simulink model "simulation_model"  (R2022a)
settings: Solver=VariableStepAuto  StartTime=0.0  StopTime=inf  FixedStep=0.02  MaxStep=0.1  RelTol=1e-3
values from neighbouring files (symbols this model uses):
  psi0 = atan(yc/xc)    [close_example.m]    (also in example_m.m)
  xc = coordinate(1)    [close_example.m]    (also in example_m.m)
  yc = coordinate(2)    [close_example.m]    (also in example_m.m)
undefined symbols (not defined in the file or in its folder): fuel_rate, gamma_pb, Pose, sigbuilder_block
libraries: simulink_extras x4, robotlib x3, simulink x1
(part 1 of 3)
settings Model: Creator=Rafal  LastModifiedBy=offroad
settings OptimizationCC: DefaultParameterBehavior=Inlined  EnhancedBackFolding=on  PassReuseOutputArgsAs=Individual arguments  ZeroExternalMemoryAtStartup=off  ZeroInternalMemoryAtStartup=off  MaxStackSize=64  OptimizeBlockOrder=speed  DifferentSizesBufferReuse=on  OptimizationCustomize=off  EfficientTunableParamExpr=on
settings DebuggingCC: ParameterTunabilityLossMsg=error
settings HardwareCC: ProdBitPerPointer=32  ProdBitPerSizeT=32  ProdBitPerPtrDiffT=32  ProdLargestAtomicFloat=None  ProdIntDivRoundTo=Undefined  ProdEndianess=Unspecified  ProdWordSize=32  ProdHWDeviceType=Generic->Unspecified (assume 32-bit Generic)  UseEmbeddedCoderFeatures=off
settings SFSimCC: MATLABDynamicMemAlloc=off
settings RTWCC: SystemTargetFile=ert.tlc  TemplateMakefile=ert_default_tmf  Toolchain=Catkin
settings CodeAppCC: ForceParamTrailComments=on  IgnoreCustomStorageClasses=off  OperatorAnnotations=on  SimulinkDataObjDesc=on  SFDataObjDesc=on  InsertBlockDesc=on
settings ERTTargetCC: SupportNonInlinedSFcns=on  ERTCustomFileTemplate=example_file_process.tlc

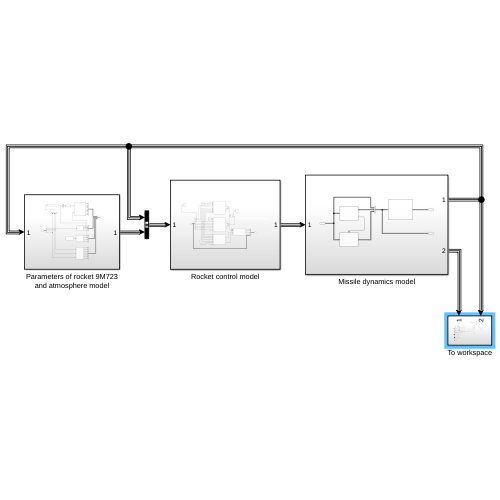
[thumbnail: Simulink's stored preview of the top-level diagram]
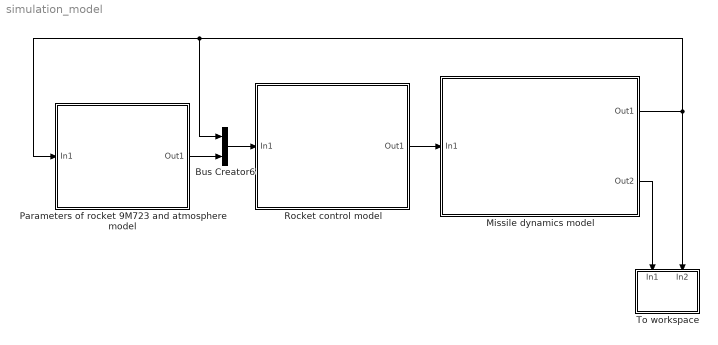
== system simulation_model ==
  Bus Creator6 : BusCreator  Inputs=2
  Missile dynamics model : Subsystem
  Parameters of rocket 9M723 and atmosphere model : Subsystem
  Rocket control model : Subsystem
  To workspace : Subsystem
  wires:
  Bus Creator6/1 -> Rocket control model/1(In1)
  Parameters of rocket 9M723 and atmosphere model/1(Out1) -> Bus Creator6/2
  Missile dynamics model/1(Out1) -> To workspace/2(In2), Parameters of rocket 9M723 and atmosphere model/1(In1), Bus Creator6/1
  Missile dynamics model/2(Out2) -> To workspace/1(In1)
  Rocket control model/1(Out1) -> Missile dynamics model/1(In1)

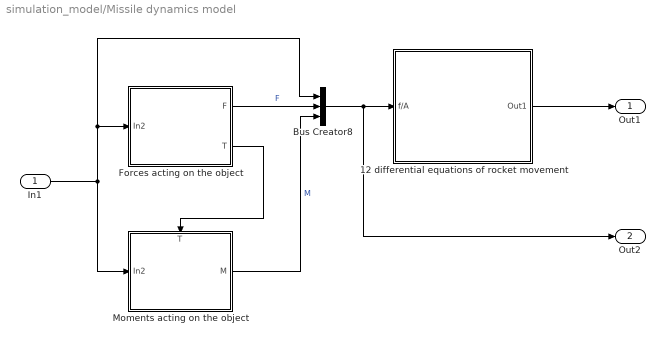
== system simulation_model/Missile dynamics model ==
  In1 : Inport
  "12 differential equations of rocket movement " : Subsystem
  Bus Creator8 : BusCreator  Inputs=3
  "Forces acting on the object " : Subsystem
  Moments acting on the object : Subsystem
      settings: PortSchema="{\"entries\":[{\"content\":{\"sides\":[{\"content\":{\"connectorIds\":[\"In1\"]},\"type\":\"ConnectorPlacement.EquallySpacedRectSide\",\"uuid\":\"23a5d515-3fe3-43ba-a5a2-a9cfb4131548\"},{\"content\":{\"connectorIds\":[\"Out1\"],\"side\":\"RIGHT\"},\"type\":\"ConnectorPlacement.EquallySpacedRectSide\",\"uuid\":\"38b37899-0e98-470d-b21c-2ca9e40fcf87\"},{\"content\":{\"connectorIds\":[\"In2\"],\"side\":\"TOP\"},\"type\":\"ConnectorPlacement.EquallySpacedRectSide\",\"uuid\":\"7a45db12-7300-424e-9c7b-41707e33aad7\"}]},\"type\":\"ConnectorPlacement.EquallySpacedConnector\",\"uuid\":\"8f829a99-de5c-4ee4-a55c-0d0490bb16ea\"}],\"packageUris\":[\"http://schema.mathworks.com/mf0/Connector/R2020b\"],\"version\":\"1.0\"}"
  Out1 : Outport
  Out2 : Outport  Port=2
  wires:
  In1/1 -> Bus Creator8/1, "Forces acting on the object "/1(In2), Moments acting on the object/1(In2)
  Bus Creator8/1 -> Out2/1, "12 differential equations of rocket movement "/1(f/A)
  Moments acting on the object/1(M) -> Bus Creator8/3  "M"
  "Forces acting on the object "/2(T) -> Moments acting on the object/2(T)
  "Forces acting on the object "/1(F) -> Bus Creator8/2  "F"
  "12 differential equations of rocket movement "/1(Out1) -> Out1/1

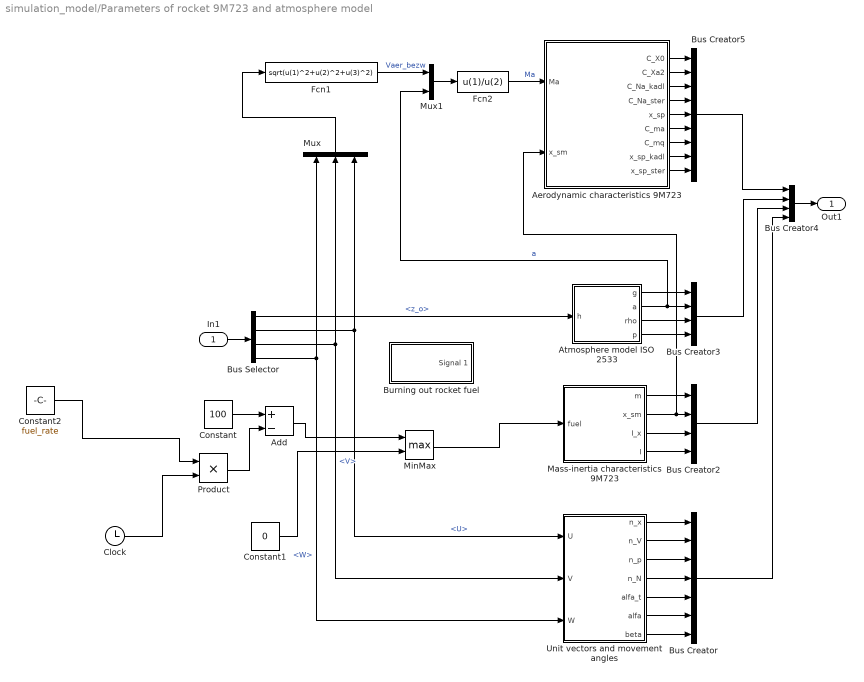
== system simulation_model/Parameters of rocket 9M723 and atmosphere model ==
  In1 : Inport
  Add : Sum  Inputs=+-
  Aerodynamic characteristics 9M723 : MATLAB Function  TreatAsAtomicUnit=on
  Atmosphere model ISO 2533 : MATLAB Function  TreatAsAtomicUnit=on
  Burning out rocket fuel : Subsystem  Tag=STV Subsys  LoadFcn=sigbuilder_block('load');  StartFcn=sigbuilder_block('start');  StopFcn=sigbuilder_block('stop');  ClipboardFcn=sigbuilder_block('clipboard');  mask(Sigbuilder block){tuvar=[0:10]}
      mask help: Simulink:masks:SigbuilderBlock_MD
      mask init:
      | if ~strcmp(get_param(bdroot(gcbh),'SimulationStatus'),'stopped') tuvar = sigbuilder_block('maskInit'); end
      settings: CopyFcn=sigbuilder_block('copy');  DeleteFcn=sigbuilder_block('delete');  ModelCloseFcn=sigbuilder_block('modelClose');  PreSaveFcn=sigbuilder_block('preSave');  PauseFcn=sigbuilder_block('pause');  ContinueFcn=sigbuilder_block('continue');  NameChangeFcn=sigbuilder_block('namechange');  OpenFcn=sigbuilder_block('open',[525 156.75 603 363.75 ]);  CloseFcn=sigbuilder_block('close');
      mask Display: plot(0, 0, 100, 100,[2, 2, 32, 32, 2], [68, 8, 8, 68, 68],[32, 2], [38, 38], [32, 19, 2],[53, 60, 44], [32, 17, 17, 2],[16, 16, 31, 31]);txt = getActiveGroup(gcbh);text(2, 100, txt,'verticalAlignment', 'top');
  Bus Creator : BusCreator  Inputs=7
  Bus Creator2 : BusCreator  Inputs=4
  Bus Creator3 : BusCreator  Inputs=4
  Bus Creator4 : BusCreator  Inputs=4
  Bus Creator5 : BusCreator  Inputs=9
  Bus Selector : BusSelector  OutputSignals=z_o,U,V,W
  Clock : Clock
  Constant : Constant  Value=100
  Constant1 : Constant  Value=0
  Constant2 : Constant  Value=fuel_rate
  Fcn1 : Fcn  Expr=sqrt(u(1)^2+u(2)^2+u(3)^2)
  Fcn2 : Fcn  Expr=u(1)/u(2)
  Mass-inertia characteristics 9M723 : MATLAB Function  TreatAsAtomicUnit=on
  MinMax : MinMax  Function=max  Inputs=2
  Mux : Mux  Inputs=3
  Mux1 : Mux  Inputs=2
  Product : Product
  Unit vectors and movement angles : MATLAB Function  TreatAsAtomicUnit=on
  Out1 : Outport
  wires:
  Aerodynamic characteristics 9M723/2(C_Xa2) -> Bus Creator5/2
  Aerodynamic characteristics 9M723/1(C_X0) -> Bus Creator5/1
  Bus Creator3/1 -> Bus Creator4/2
  Atmosphere model ISO 2533/2(a) -> Mux1/2, Bus Creator3/2  "a"
  Aerodynamic characteristics 9M723/5(x_sp) -> Bus Creator5/5
  Aerodynamic characteristics 9M723/4(C_Na_ster) -> Bus Creator5/4
  Aerodynamic characteristics 9M723/9(x_sp_ster) -> Bus Creator5/9
  Aerodynamic characteristics 9M723/8(x_sp_kadl) -> Bus Creator5/8
  Mass-inertia characteristics 9M723/3(I_x) -> Bus Creator2/3
  Bus Creator5/1 -> Bus Creator4/1
  Unit vectors and movement angles/4(n_N) -> Bus Creator/4
  Mux/1 -> Fcn1/1
  Aerodynamic characteristics 9M723/3(C_Na_kadl) -> Bus Creator5/3
  Mass-inertia characteristics 9M723/4(I) -> Bus Creator2/4
  Bus Creator/1 -> Bus Creator4/4
  Bus Selector/1 -> Atmosphere model ISO 2533/1(h)  "<z_o>"
  Bus Creator4/1 -> Out1/1
  Fcn1/1 -> Mux1/1  "Vaer_bezw"
  Unit vectors and movement angles/7(beta) -> Bus Creator/7
  Bus Selector/4 -> Mux/1, Unit vectors and movement angles/3(W)  "<W>"
  Atmosphere model ISO 2533/1(g) -> Bus Creator3/1
  Bus Selector/3 -> Mux/2, Unit vectors and movement angles/2(V)  "<V>"
  Unit vectors and movement angles/6(alfa) -> Bus Creator/6
  Unit vectors and movement angles/3(n_p) -> Bus Creator/3
  Unit vectors and movement angles/2(n_V) -> Bus Creator/2
  Unit vectors and movement angles/1(n_x) -> Bus Creator/1
  Unit vectors and movement angles/5(alfa_t) -> Bus Creator/5
  Bus Creator2/1 -> Bus Creator4/3
  Bus Selector/2 -> Unit vectors and movement angles/1(U), Mux/3  "<U>"
  Fcn2/1 -> Aerodynamic characteristics 9M723/1(Ma)  "Ma"
  Mass-inertia characteristics 9M723/1(m) -> Bus Creator2/1
  Mass-inertia characteristics 9M723/2(x_sm) -> Aerodynamic characteristics 9M723/2(x_sm), Bus Creator2/2
  Aerodynamic characteristics 9M723/6(C_ma) -> Bus Creator5/6
  Aerodynamic characteristics 9M723/7(C_mq) -> Bus Creator5/7
  Atmosphere model ISO 2533/4(p) -> Bus Creator3/4
  Mux1/1 -> Fcn2/1
  Atmosphere model ISO 2533/3(rho) -> Bus Creator3/3
  In1/1 -> Bus Selector/1
  Clock/1 -> Product/2
  Constant/1 -> Add/1
  Product/1 -> Add/2
  Add/1 -> MinMax/1
  Constant1/1 -> MinMax/2
  MinMax/1 -> Mass-inertia characteristics 9M723/1(fuel)
  Constant2/1 -> Product/1

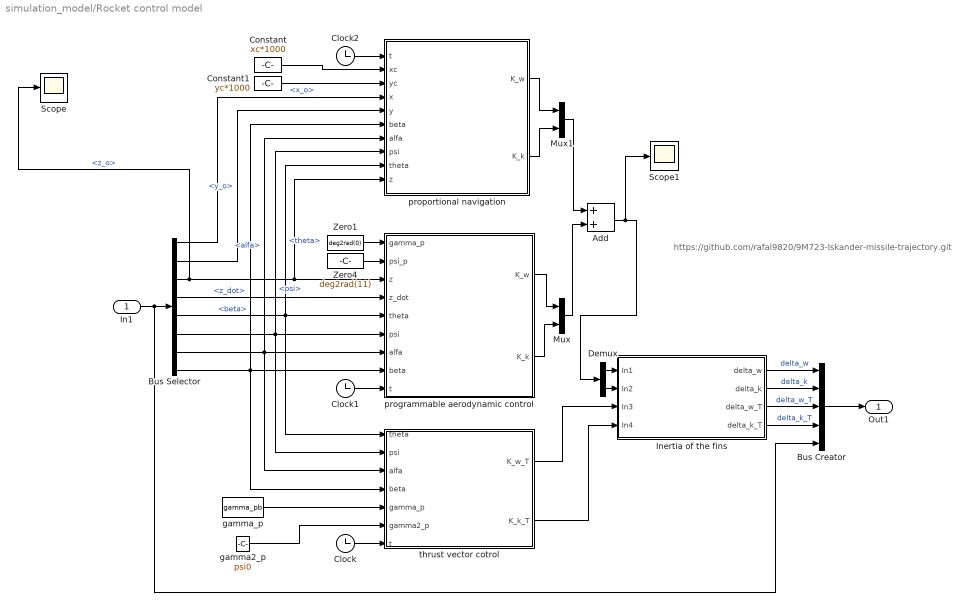
== system simulation_model/Rocket control model ==
  note: https://github.com/rafal9820/9M723-Iskander-missile-trajectory.git
  In1 : Inport
  Add : Sum
  Bus Creator : BusCreator  Inputs=5
  Bus Selector : BusSelector  OutputSignals=signal1.x_o,signal1.y_o,signal1.z_o,signal1.z_dot,signal1.theta,signal1.psi,signal2.signal4.alfa,signal2.signal4.beta
  Clock : Clock
  Clock1 : Clock
  Clock2 : Clock
  Constant : Constant  Value=xc*1000
  Constant1 : Constant  Value=yc*1000
  Demux : Demux  Outputs=2
  "Inertia of the fins " : Subsystem
  Mux : Mux  Inputs=2
  Mux1 : Mux  Inputs=2
  Scope : Scope
  Scope1 : Scope
  Zero1 : Constant  Value=deg2rad(0)  OutDataTypeStr=Inherit: Inherit via back propagation
  Zero4 : Constant  Value=deg2rad(11)  OutDataTypeStr=Inherit: Inherit via back propagation
  gamma2_p : Constant  Value=psi0  OutDataTypeStr=Inherit: Inherit via back propagation
  gamma_p : Constant  Value=gamma_pb  OutDataTypeStr=Inherit: Inherit via back propagation
  programmable aerodynamic control : MATLAB Function  TreatAsAtomicUnit=on
  proportional navigation : MATLAB Function  TreatAsAtomicUnit=on
  thrust vector cotrol : MATLAB Function  TreatAsAtomicUnit=on
  Out1 : Outport
  wires:
  In1/1 -> Bus Selector/1, Bus Creator/5
  Bus Creator/1 -> Out1/1
  Bus Selector/5 -> programmable aerodynamic control/5(theta), proportional navigation/9(theta), thrust vector cotrol/1(theta)  "<theta>"
  Bus Selector/6 -> thrust vector cotrol/2(psi), programmable aerodynamic control/6(psi), proportional navigation/8(psi)  "<psi>"
  Clock/1 -> thrust vector cotrol/7(t)
  Clock1/1 -> programmable aerodynamic control/9(t)
  Zero4/1 -> programmable aerodynamic control/2(psi_p)
  Zero1/1 -> programmable aerodynamic control/1(gamma_p)
  Bus Selector/7 -> proportional navigation/7(alfa), programmable aerodynamic control/7(alfa), thrust vector cotrol/3(alfa)  "<alfa>"
  Bus Selector/8 -> proportional navigation/6(beta), programmable aerodynamic control/8(beta), thrust vector cotrol/4(beta)  "<beta>"
  gamma2_p/1 -> thrust vector cotrol/6(gamma2_p)
  thrust vector cotrol/1(K_w_T) -> "Inertia of the fins "/3(In3)
  thrust vector cotrol/2(K_k_T) -> "Inertia of the fins "/4(In4)
  "Inertia of the fins "/1(delta_w) -> Bus Creator/1  "delta_w"
  "Inertia of the fins "/2(delta_k) -> Bus Creator/2  "delta_k"
  "Inertia of the fins "/3(delta_w_T) -> Bus Creator/3  "delta_w_T"
  "Inertia of the fins "/4(delta_k_T) -> Bus Creator/4  "delta_k_T"
  Bus Selector/3 -> Scope/1, programmable aerodynamic control/3(z), proportional navigation/10(z)  "<z_o>"
  Bus Selector/4 -> programmable aerodynamic control/4(z_dot)  "<z_dot>"
  gamma_p/1 -> thrust vector cotrol/5(gamma_p)
  Bus Selector/1 -> proportional navigation/4(x)  "<x_o>"
  Bus Selector/2 -> proportional navigation/5(y)  "<y_o>"
  Constant/1 -> proportional navigation/2(xc)
  Constant1/1 -> proportional navigation/3(yc)
  Demux/1 -> "Inertia of the fins "/1(In1)
  Demux/2 -> "Inertia of the fins "/2(In2)
  programmable aerodynamic control/2(K_k) -> Mux/2
  programmable aerodynamic control/1(K_w) -> Mux/1
  proportional navigation/1(K_w) -> Mux1/1
  proportional navigation/2(K_k) -> Mux1/2
  Clock2/1 -> proportional navigation/1(t)
  Add/1 -> Scope1/1, Demux/1
  Mux1/1 -> Add/1
  Mux/1 -> Add/2

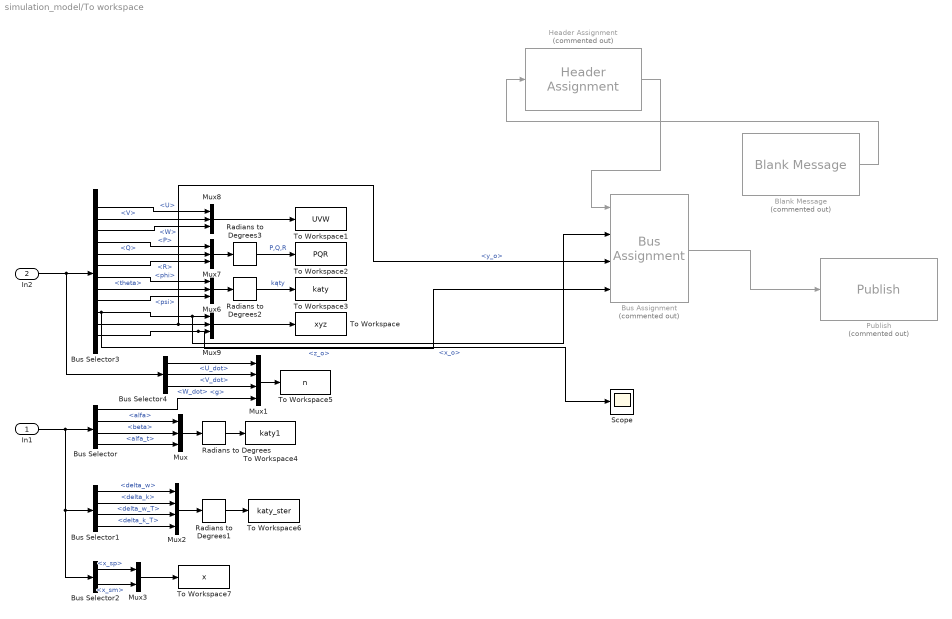
== system simulation_model/To workspace ==
  In1 : Inport
  In2 : Inport  Port=2
  Blank Message : robotlib/Blank Message  Commented=on  messageClass=Message  entityType=nav_msgs/Odometry  messageType=nav_msgs/Odometry  SampleTime=inf  legacyBusStruct=off
  Bus Assignment : BusAssignment  Commented=on  AssignedSignals=Pose.Pose.Position.X,Pose.Pose.Position.Y,Pose.Pose.Position.Z
  Bus Selector : BusSelector  OutputSignals=signal1.signal5.signal2.signal2.g,signal1.signal5.signal2.signal4.alfa,signal1.signal5.signal2.signal4.beta,signal1.signal5.signal2.signal4.alfa_t
  Bus Selector1 : BusSelector  OutputSignals=signal1.delta_w,signal1.delta_k,signal1.delta_w_T,signal1.delta_k_T
  Bus Selector2 : BusSelector  OutputSignals=signal1.signal5.signal2.signal1.x_sp,signal1.signal5.signal2.signal3.x_sm
  Bus Selector3 : BusSelector  OutputSignals=U,V,W,P,Q,R,phi,theta,psi,x_o,y_o,z_o
  Bus Selector4 : BusSelector  OutputSignals=U_dot,V_dot,W_dot
  Header Assignment : robotlib/Header Assignment  Commented=on  SetFrameID=on  FrameID=map  InsertTimeStamp=on  SetHeaderFieldName=Use the default Header field name  HeaderFieldName=Header
      settings: SourceProductBaseCode=RR
  Mux{,6..9} (5 alike) : Mux  Inputs=3
  Mux1 : Mux
  Mux2 : Mux
  Mux3 : Mux  Inputs=2
  Publish : robotlib/Publish  Commented=on  topicSource=Specify your own  topic=/my_topic  messageType=nav_msgs/Odometry  legacyBusStruct=off  messageQueueLength=1
  Radians to Degrees{,1..3} (4 alike) : simulink_extras/Transformations/Radians to Degrees
  Scope : Scope
  To Workspace : ToWorkspace  VariableName=xyz  SaveFormat=Timeseries  SampleTime=-1
  To Workspace1 : ToWorkspace  VariableName=UVW  SaveFormat=Timeseries  SampleTime=-1
  To Workspace2 : ToWorkspace  VariableName=PQR  SaveFormat=Timeseries  SampleTime=-1
  To Workspace3 : ToWorkspace  VariableName=katy  SaveFormat=Timeseries  SampleTime=-1
  To Workspace4 : ToWorkspace  VariableName=katy1  SaveFormat=Timeseries  SampleTime=-1
  To Workspace5 : ToWorkspace  VariableName=n  SaveFormat=Timeseries  SampleTime=-1
  To Workspace6 : ToWorkspace  VariableName=katy_ster  SaveFormat=Timeseries  SampleTime=-1
  To Workspace7 : ToWorkspace  VariableName=x  SaveFormat=Timeseries  SampleTime=-1
  wires:
  Mux8/1 -> To Workspace1/1
  Mux7/1 -> Radians to Degrees3/1
  Bus Selector4/1 -> Mux1/1  "<U_dot>"
  Bus Selector4/2 -> Mux1/2  "<V_dot>"
  Radians to Degrees2/1 -> To Workspace3/1  "kąty"
  Radians to Degrees3/1 -> To Workspace2/1  "P,Q,R"
  Bus Selector3/9 -> Mux6/3  "<psi>"
  Bus Selector/1 -> Mux1/4  "<g>"
  Bus Selector/4 -> Mux/3  "<alfa_t>"
  Bus Selector3/8 -> Mux6/2  "<theta>"
  Bus Selector3/7 -> Mux6/1  "<phi>"
  Bus Selector4/3 -> Mux1/3  "<W_dot>"
  Mux6/1 -> Radians to Degrees2/1
  Mux9/1 -> To Workspace/1
  Bus Selector3/11 -> Bus Assignment/3, Mux9/2  "<y_o>"
  Bus Selector3/12 -> Bus Assignment/4, Mux9/3  "<z_o>"
  Bus Selector3/10 -> Scope/1, Bus Assignment/2, Mux9/1  "<x_o>"
  Bus Selector3/3 -> Mux8/3  "<W>"
  Bus Selector3/2 -> Mux8/2  "<V>"
  Bus Selector3/5 -> Mux7/2  "<Q>"
  Bus Selector3/4 -> Mux7/1  "<P>"
  Bus Selector3/6 -> Mux7/3  "<R>"
  Bus Selector/2 -> Mux/1  "<alfa>"
  Mux1/1 -> To Workspace5/1
  Bus Selector/3 -> Mux/2  "<beta>"
  Bus Selector3/1 -> Mux8/1  "<U>"
  Mux/1 -> Radians to Degrees/1
  Radians to Degrees/1 -> To Workspace4/1
  In2/1 -> Bus Selector4/1, Bus Selector3/1
  In1/1 -> Bus Selector2/1, Bus Selector1/1, Bus Selector/1
  Bus Selector1/2 -> Mux2/2  "<delta_k>"
  Bus Selector1/1 -> Mux2/1  "<delta_w>"
  Bus Selector1/3 -> Mux2/3  "<delta_w_T>"
  Bus Selector1/4 -> Mux2/4  "<delta_k_T>"
  Mux2/1 -> Radians to Degrees1/1
  Radians to Degrees1/1 -> To Workspace6/1
  Bus Selector2/1 -> Mux3/1  "<x_sp>"
  Bus Selector2/2 -> Mux3/2  "<x_sm>"
  Mux3/1 -> To Workspace7/1
  Blank Message/1 -> Header Assignment/1
  Bus Assignment/1 -> Publish/1
  Header Assignment/1 -> Bus Assignment/1

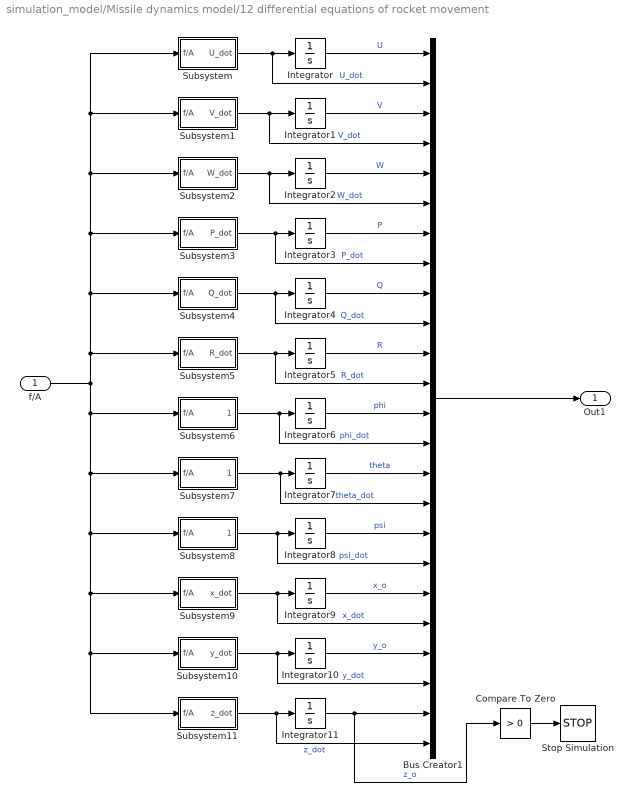
== system simulation_model/Missile dynamics model/12 differential equations of rocket movement  ==
  f/A : Inport
  Bus Creator1 : BusCreator  Inputs=24
  Compare To Zero : simulink/Logic and Bit Operations/Compare To Zero  relop=>  OutDataTypeStr=boolean
  Integrator : Integrator  InitialCondition=0.000001
  Integrator{1..6,9..11} (9 alike) : Integrator
  Integrator7 : Integrator  InitialCondition=deg2rad(90)
  Integrator8 : Integrator  InitialCondition=psi0
  Stop Simulation : Stop
  Subsystem : Subsystem
  Subsystem1 : Subsystem
  Subsystem10 : Subsystem
  Subsystem11 : Subsystem
  Subsystem2 : Subsystem
  Subsystem3 : Subsystem
  Subsystem4 : Subsystem
  Subsystem5 : Subsystem
  Subsystem6 : Subsystem
  Subsystem7 : Subsystem
  Subsystem8 : Subsystem
  Subsystem9 : Subsystem
  Out1 : Outport
  wires:
  Integrator4/1 -> Bus Creator1/9  "Q"
  Subsystem11/1(z_dot) -> Bus Creator1/24, Integrator11/1  "z_dot"
  Subsystem3/1(P_dot) -> Bus Creator1/8, Integrator3/1  "P_dot"
  Subsystem7/1(theta_dot) -> Bus Creator1/16, Integrator7/1  "theta_dot"
  Integrator10/1 -> Bus Creator1/21  "y_o"
  Compare To Zero/1 -> Stop Simulation/1
  Subsystem4/1(Q_dot) -> Bus Creator1/10, Integrator4/1  "Q_dot"
  f/A/1 -> Subsystem3/1(f/A), Subsystem2/1(f/A), Subsystem1/1(f/A), Subsystem/1(f/A), Subsystem4/1(f/A), Subsystem5/1(f/A), Subsystem11/1(f/A), Subsystem10/1(f/A), Subsystem9/1(f/A), Subsystem8/1(f/A), Subsystem7/1(f/A), Subsystem6/1(f/A)
  Subsystem6/1(phi_dot) -> Integrator6/1, Bus Creator1/14  "phi_dot"
  Integrator8/1 -> Bus Creator1/17  "psi"
  Subsystem1/1(V_dot) -> Bus Creator1/4, Integrator1/1  "V_dot"
  Subsystem9/1(x_dot) -> Bus Creator1/20, Integrator9/1  "x_dot"
  Integrator9/1 -> Bus Creator1/19  "x_o"
  Integrator11/1 -> Bus Creator1/23, Compare To Zero/1  "z_o"
  Integrator2/1 -> Bus Creator1/5  "W"
  Subsystem2/1(W_dot) -> Bus Creator1/6, Integrator2/1  "W_dot"
  Integrator3/1 -> Bus Creator1/7  "P"
  Subsystem8/1(psi_dot) -> Bus Creator1/18, Integrator8/1  "psi_dot"
  Bus Creator1/1 -> Out1/1
  Subsystem10/1(y_dot) -> Bus Creator1/22, Integrator10/1  "y_dot"
  Subsystem/1(U_dot) -> Bus Creator1/2, Integrator/1  "U_dot"
  Subsystem5/1(R_dot) -> Bus Creator1/12, Integrator5/1  "R_dot"
  Integrator5/1 -> Bus Creator1/11  "R"
  Integrator/1 -> Bus Creator1/1  "U"
  Integrator1/1 -> Bus Creator1/3  "V"
  Integrator7/1 -> Bus Creator1/15  "theta"
  Integrator6/1 -> Bus Creator1/13  "phi"

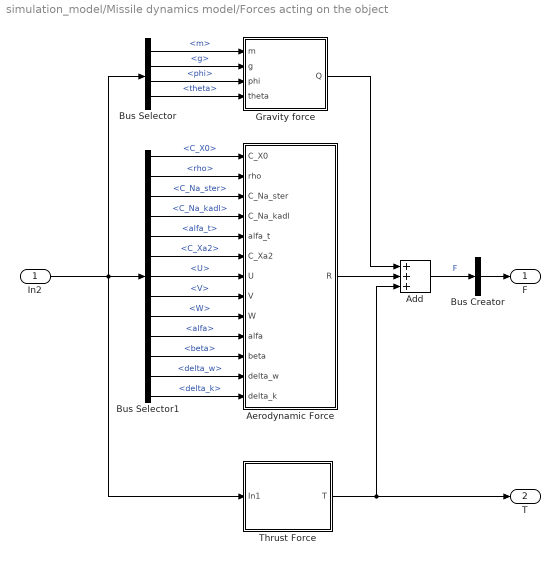
== system simulation_model/Missile dynamics model/Forces acting on the object  ==
  In2 : Inport
  Add : Sum  Inputs=+++
  Aerodynamic Force : MATLAB Function  TreatAsAtomicUnit=on
  Bus Creator : BusCreator  Inputs=1
  Bus Selector : BusSelector  OutputSignals=signal5.signal2.signal3.m,signal5.signal2.signal2.g,signal5.signal1.phi,signal5.signal1.theta
  Bus Selector1 : BusSelector  OutputSignals=signal5.signal2.signal1.C_X0,signal5.signal2.signal2.rho,signal5.signal2.signal1.C_Na_ster,signal5.signal2.signal1.C_Na_kadl,signal5.signal2.signal4.alfa_t,signal5.signal2.signal1.C_Xa2,signal5.signal1.U,signal5.signal1.V,signal5.signal1.W,signal5.signal2.signal4.alfa,signal5.signal2.signal4.beta,delta_w,delta_k
  Gravity force : MATLAB Function  TreatAsAtomicUnit=on
  Thrust Force : Subsystem
  F : Outport
  T : Outport  Port=2
  wires:
  In2/1 -> Bus Selector/1, Thrust Force/1(In1), Bus Selector1/1
  Bus Selector/1 -> Gravity force/1(m)  "<m>"
  Bus Selector/2 -> Gravity force/2(g)  "<g>"
  Bus Selector1/1 -> Aerodynamic Force/1(C_X0)  "<C_X0>"
  Bus Selector1/2 -> Aerodynamic Force/2(rho)  "<rho>"
  Bus Selector1/3 -> Aerodynamic Force/3(C_Na_ster)  "<C_Na_ster>"
  Bus Selector1/4 -> Aerodynamic Force/4(C_Na_kadl)  "<C_Na_kadl>"
  Bus Selector1/5 -> Aerodynamic Force/5(alfa_t)  "<alfa_t>"
  Bus Selector1/6 -> Aerodynamic Force/6(C_Xa2)  "<C_Xa2>"
  Bus Selector1/10 -> Aerodynamic Force/10(alfa)  "<alfa>"
  Bus Selector1/11 -> Aerodynamic Force/11(beta)  "<beta>"
  Gravity force/1(Q) -> Add/1
  Add/1 -> Bus Creator/1  "F"
  Bus Creator/1 -> F/1
  Bus Selector/3 -> Gravity force/3(phi)  "<phi>"
  Bus Selector/4 -> Gravity force/4(theta)  "<theta>"
  Bus Selector1/7 -> Aerodynamic Force/7(U)  "<U>"
  Bus Selector1/8 -> Aerodynamic Force/8(V)  "<V>"
  Bus Selector1/9 -> Aerodynamic Force/9(W)  "<W>"
  Thrust Force/1(T) -> T/1, Add/3
  Bus Selector1/12 -> Aerodynamic Force/12(delta_w)  "<delta_w>"
  Bus Selector1/13 -> Aerodynamic Force/13(delta_k)  "<delta_k>"
  Aerodynamic Force/1(R) -> Add/2

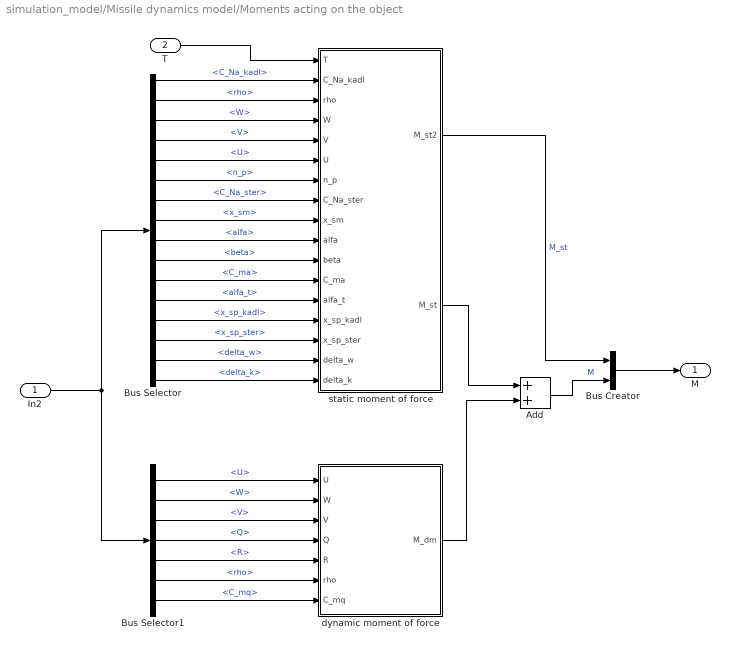
== system simulation_model/Missile dynamics model/Moments acting on the object ==
  In2 : Inport
  T : Inport  Port=2
  Add : Sum
  Bus Creator : BusCreator  Inputs=2
  Bus Selector : BusSelector  OutputSignals=signal5.signal2.signal1.C_Na_kadl,signal5.signal2.signal2.rho,signal5.signal1.W,signal5.signal1.V,signal5.signal1.U,signal5.signal2.signal4.n_p,signal5.signal2.signal1.C_Na_ster,signal5.signal2.signal3.x_sm,signal5.signal2.signal4.alfa,signal5.signal2.signal4.beta,signal5.signal2.signal1.C_ma,signal5.signal2.signal4.alfa_t,signal5.signal2.signal1.x_sp_kadl,signal5.signal2.signal1.x_sp_ster,delta_w,delta_k
  Bus Selector1 : BusSelector  OutputSignals=signal5.signal1.U,signal5.signal1.W,signal5.signal1.V,signal5.signal1.Q,signal5.signal1.R,signal5.signal2.signal2.rho,signal5.signal2.signal1.C_mq
  dynamic moment of force : MATLAB Function  TreatAsAtomicUnit=on
  static moment of force : MATLAB Function  TreatAsAtomicUnit=on
  M : Outport
  wires:
  In2/1 -> Bus Selector/1, Bus Selector1/1
  Bus Selector/1 -> static moment of force/2(C_Na_kadl)  "<C_Na_kadl>"
  Bus Selector/7 -> static moment of force/8(C_Na_ster)  "<C_Na_ster>"
  Bus Selector/8 -> static moment of force/9(x_sm)  "<x_sm>"
  Bus Selector/9 -> static moment of force/10(alfa)  "<alfa>"
  Bus Selector/10 -> static moment of force/11(beta)  "<beta>"
  Bus Selector1/6 -> dynamic moment of force/6(rho)  "<rho>"
  Bus Selector1/7 -> dynamic moment of force/7(C_mq)  "<C_mq>"
  Add/1 -> Bus Creator/2  "M"
  Bus Creator/1 -> M/1
  Bus Selector1/4 -> dynamic moment of force/4(Q)  "<Q>"
  Bus Selector1/5 -> dynamic moment of force/5(R)  "<R>"
  Bus Selector1/3 -> dynamic moment of force/3(V)  "<V>"
  Bus Selector1/2 -> dynamic moment of force/2(W)  "<W>"
  Bus Selector1/1 -> dynamic moment of force/1(U)  "<U>"
  Bus Selector/3 -> static moment of force/4(W)  "<W>"
  Bus Selector/4 -> static moment of force/5(V)  "<V>"
  Bus Selector/5 -> static moment of force/6(U)  "<U>"
  Bus Selector/6 -> static moment of force/7(n_p)  "<n_p>"
  Bus Selector/2 -> static moment of force/3(rho)  "<rho>"
  Bus Selector/11 -> static moment of force/12(C_ma)  "<C_ma>"
  static moment of force/1(M_st2) -> Bus Creator/1  "M_st"
  Bus Selector/12 -> static moment of force/13(alfa_t)  "<alfa_t>"
  Bus Selector/13 -> static moment of force/14(x_sp_kadl)  "<x_sp_kadl>"
  Bus Selector/14 -> static moment of force/15(x_sp_ster)  "<x_sp_ster>"
  T/1 -> static moment of force/1(T)
  Bus Selector/15 -> static moment of force/16(delta_w)  "<delta_w>"
  Bus Selector/16 -> static moment of force/17(delta_k)  "<delta_k>"
  dynamic moment of force/1(M_dm) -> Add/2
  static moment of force/2(M_st) -> Add/1

== system simulation_model/Parameters of rocket 9M723 and atmosphere model/Burning out rocket fuel ==
  Demux : Demux  Tag=STV Demux  Outputs=1
      settings: DisplayOption=none
  FromWs : FromWorkspace  Tag=STV FromWs  VariableName=tuvar
      SigBuilderData=|
      | common.afterFinalStr = 'Extrapolate'
      | common.sampleTime = 0
      | dataSet.timeRange = [0 1000]
      | dataSet.name = 'Group 1'
      | sbobj.Groups.Name = 'Group 1'
      | sbobj.Groups.Signals.Name = 'Signal 1'
      | sbobj.Groups.Signals.XData = [0 1 49.5 1000]
      | sbobj.Groups.Signals.YData = [97.5 94 0 0.5]
      | sbobj.Groups.TimeRange = [0 1000]
  Signal 1 : Outport  Tag=STV Outport
  wires:
  FromWs/1 -> Demux/1
  Demux/1 -> Signal 1/1

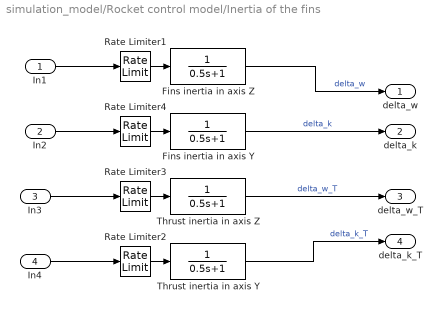
== system simulation_model/Rocket control model/Inertia of the fins  ==
  In1 : Inport
  In2 : Inport  Port=2
  In3 : Inport  Port=3
  In4 : Inport  Port=4
  Fins inertia in axis Y : TransferFcn  Denominator=[0.5 1]
  Fins inertia in axis Z : TransferFcn  Denominator=[0.5 1]
  Rate Limiter1 : RateLimiter  RisingSlewLimit=deg2rad(3.2)  FallingSlewLimit=deg2rad(-2.2)  SampleTimeMode=inherited
  Rate Limiter2 : RateLimiter  RisingSlewLimit=deg2rad(0.00005)  FallingSlewLimit=deg2rad(-0.00005)  SampleTimeMode=inherited
  Rate Limiter3 : RateLimiter  RisingSlewLimit=deg2rad(0.2)  FallingSlewLimit=deg2rad(-0.2)  SampleTimeMode=inherited
  Rate Limiter4 : RateLimiter  RisingSlewLimit=deg2rad(1.8)  FallingSlewLimit=deg2rad(-1.8)  SampleTimeMode=inherited
  Thrust inertia in axis Y : TransferFcn  Denominator=[0.5 1]
  Thrust inertia in axis Z : TransferFcn  Denominator=[0.5 1]
  delta_w : Outport
  delta_k : Outport  Port=2
  delta_w_T : Outport  Port=3
  delta_k_T : Outport  Port=4
  wires:
  Thrust inertia in axis Z/1 -> delta_w_T/1  "delta_w_T"
  Fins inertia in axis Z/1 -> delta_w/1  "delta_w"
  Fins inertia in axis Y/1 -> delta_k/1  "delta_k"
  Thrust inertia in axis Y/1 -> delta_k_T/1  "delta_k_T"
  Rate Limiter1/1 -> Fins inertia in axis Z/1
  In2/1 -> Rate Limiter4/1
  Rate Limiter3/1 -> Thrust inertia in axis Z/1
  Rate Limiter2/1 -> Thrust inertia in axis Y/1
  In4/1 -> Rate Limiter2/1
  In1/1 -> Rate Limiter1/1
  In3/1 -> Rate Limiter3/1
  Rate Limiter4/1 -> Fins inertia in axis Y/1

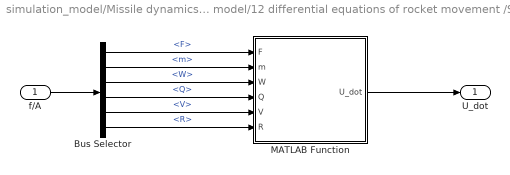
== system simulation_model/Missile dynamics model/12 differential equations of rocket movement /Subsystem ==
  f/A : Inport
  Bus Selector : BusSelector  OutputSignals=F.F,signal1.signal5.signal2.signal3.m,signal1.signal5.signal1.W,signal1.signal5.signal1.Q,signal1.signal5.signal1.V,signal1.signal5.signal1.R
  MATLAB Function : MATLAB Function  TreatAsAtomicUnit=on
  U_dot : Outport
  wires:
  f/A/1 -> Bus Selector/1
  Bus Selector/1 -> MATLAB Function/1(F)  "<F>"
  Bus Selector/2 -> MATLAB Function/2(m)  "<m>"
  Bus Selector/3 -> MATLAB Function/3(W)  "<W>"
  Bus Selector/4 -> MATLAB Function/4(Q)  "<Q>"
  Bus Selector/5 -> MATLAB Function/5(V)  "<V>"
  Bus Selector/6 -> MATLAB Function/6(R)  "<R>"
  MATLAB Function/1(U_dot) -> U_dot/1

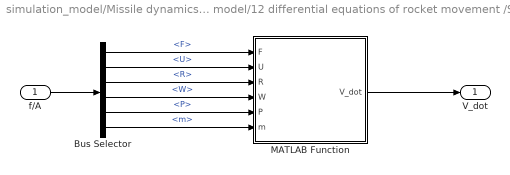
== system simulation_model/Missile dynamics model/12 differential equations of rocket movement /Subsystem1 ==
  f/A : Inport
  Bus Selector : BusSelector  OutputSignals=F.F,signal1.signal5.signal1.U,signal1.signal5.signal1.R,signal1.signal5.signal1.W,signal1.signal5.signal1.P,signal1.signal5.signal2.signal3.m
  MATLAB Function : MATLAB Function  TreatAsAtomicUnit=on
  V_dot : Outport
  wires:
  f/A/1 -> Bus Selector/1
  Bus Selector/1 -> MATLAB Function/1(F)  "<F>"
  Bus Selector/2 -> MATLAB Function/2(U)  "<U>"
  Bus Selector/3 -> MATLAB Function/3(R)  "<R>"
  Bus Selector/4 -> MATLAB Function/4(W)  "<W>"
  Bus Selector/5 -> MATLAB Function/5(P)  "<P>"
  Bus Selector/6 -> MATLAB Function/6(m)  "<m>"
  MATLAB Function/1(V_dot) -> V_dot/1

== system simulation_model/Missile dynamics model/12 differential equations of rocket movement /Subsystem10 ==
  f/A : Inport
  Bus Selector : BusSelector  OutputSignals=signal1.signal5.signal1.U,signal1.signal5.signal1.V,signal1.signal5.signal1.W,signal1.signal5.signal1.theta,signal1.signal5.signal1.phi,signal1.signal5.signal1.psi
  MATLAB Function : MATLAB Function  TreatAsAtomicUnit=on
  y_dot : Outport
  wires:
  MATLAB Function/1(y_dot) -> y_dot/1
  Bus Selector/6 -> MATLAB Function/6(psi)  "<psi>"
  Bus Selector/5 -> MATLAB Function/5(phi)  "<phi>"
  Bus Selector/4 -> MATLAB Function/4(theta)  "<theta>"
  Bus Selector/3 -> MATLAB Function/3(W)  "<W>"
  Bus Selector/2 -> MATLAB Function/2(V)  "<V>"
  Bus Selector/1 -> MATLAB Function/1(U)  "<U>"
  f/A/1 -> Bus Selector/1

== system simulation_model/Missile dynamics model/12 differential equations of rocket movement /Subsystem11 ==
  f/A : Inport
  Bus Selector : BusSelector  OutputSignals=signal1.signal5.signal1.U,signal1.signal5.signal1.V,signal1.signal5.signal1.W,signal1.signal5.signal1.theta,signal1.signal5.signal1.phi
  MATLAB Function : MATLAB Function  TreatAsAtomicUnit=on
  z_dot : Outport
  wires:
  f/A/1 -> Bus Selector/1
  Bus Selector/1 -> MATLAB Function/1(U)  "<U>"
  Bus Selector/2 -> MATLAB Function/2(V)  "<V>"
  Bus Selector/3 -> MATLAB Function/3(W)  "<W>"
  Bus Selector/4 -> MATLAB Function/4(theta)  "<theta>"
  Bus Selector/5 -> MATLAB Function/5(phi)  "<phi>"
  MATLAB Function/1(z_dot) -> z_dot/1

== system simulation_model/Missile dynamics model/12 differential equations of rocket movement /Subsystem2 ==
  f/A : Inport
  Bus Selector : BusSelector  OutputSignals=F.F,signal1.signal5.signal2.signal3.m,signal1.signal5.signal1.U,signal1.signal5.signal1.Q,signal1.signal5.signal1.V,signal1.signal5.signal1.P
  MATLAB Function : MATLAB Function  TreatAsAtomicUnit=on
  W_dot : Outport
  wires:
  f/A/1 -> Bus Selector/1
  Bus Selector/1 -> MATLAB Function/1(F)  "<F>"
  Bus Selector/2 -> MATLAB Function/2(m)  "<m>"
  Bus Selector/3 -> MATLAB Function/3(U)  "<U>"
  Bus Selector/4 -> MATLAB Function/4(Q)  "<Q>"
  Bus Selector/5 -> MATLAB Function/5(V)  "<V>"
  Bus Selector/6 -> MATLAB Function/6(P)  "<P>"
  MATLAB Function/1(W_dot) -> W_dot/1

== system simulation_model/Missile dynamics model/12 differential equations of rocket movement /Subsystem3 ==
  f/A : Inport
  Bus Selector : BusSelector  OutputSignals=M.M,signal1.signal5.signal2.signal3.I_x
  MATLAB Function : MATLAB Function  TreatAsAtomicUnit=on
  P_dot : Outport
  wires:
  f/A/1 -> Bus Selector/1
  Bus Selector/1 -> MATLAB Function/1(M)  "<M>"
  Bus Selector/2 -> MATLAB Function/2(I_x)  "<I_x>"
  MATLAB Function/1(P_dot) -> P_dot/1

== system simulation_model/Missile dynamics model/12 differential equations of rocket movement /Subsystem4 ==
  f/A : Inport
  Bus Selector : BusSelector  OutputSignals=M.M,signal1.signal5.signal1.P,signal1.signal5.signal1.R,signal1.signal5.signal2.signal3.I,signal1.signal5.signal2.signal3.I_x
  MATLAB Function : MATLAB Function  TreatAsAtomicUnit=on
  Q_dot : Outport
  wires:
  f/A/1 -> Bus Selector/1
  Bus Selector/2 -> MATLAB Function/2(P)  "<P>"
  Bus Selector/3 -> MATLAB Function/3(R)  "<R>"
  Bus Selector/4 -> MATLAB Function/4(I)  "<I>"
  Bus Selector/5 -> MATLAB Function/5(I_x)  "<I_x>"
  Bus Selector/1 -> MATLAB Function/1(M)  "<M>"
  MATLAB Function/1(Q_dot) -> Q_dot/1

== system simulation_model/Missile dynamics model/12 differential equations of rocket movement /Subsystem5 ==
  f/A : Inport
  Bus Selector : BusSelector  OutputSignals=M.M,signal1.signal5.signal1.P,signal1.signal5.signal1.Q,signal1.signal5.signal2.signal3.I,signal1.signal5.signal2.signal3.I_x
  MATLAB Function : MATLAB Function  TreatAsAtomicUnit=on
  R_dot : Outport
  wires:
  f/A/1 -> Bus Selector/1
  Bus Selector/2 -> MATLAB Function/2(P)  "<P>"
  Bus Selector/3 -> MATLAB Function/3(Q)  "<Q>"
  Bus Selector/4 -> MATLAB Function/4(I)  "<I>"
  Bus Selector/5 -> MATLAB Function/5(I_x)  "<I_x>"
  Bus Selector/1 -> MATLAB Function/1(M)  "<M>"
  MATLAB Function/1(R_dot) -> R_dot/1

== system simulation_model/Missile dynamics model/12 differential equations of rocket movement /Subsystem6 ==
  f/A : Inport
  Bus Selector : BusSelector  OutputSignals=signal1.signal5.signal1.P,signal1.signal5.signal1.Q,signal1.signal5.signal1.phi,signal1.signal5.signal1.R,signal1.signal5.signal1.theta
  MATLAB Function : MATLAB Function  TreatAsAtomicUnit=on
  phi_dot : Outport
  wires:
  f/A/1 -> Bus Selector/1
  Bus Selector/1 -> MATLAB Function/1(P)  "<P>"
  Bus Selector/2 -> MATLAB Function/2(Q)  "<Q>"
  Bus Selector/3 -> MATLAB Function/3(phi)  "<phi>"
  Bus Selector/4 -> MATLAB Function/4(R)  "<R>"
  Bus Selector/5 -> MATLAB Function/5(theta)  "<theta>"
  MATLAB Function/1(phi_dot) -> phi_dot/1

== system simulation_model/Missile dynamics model/12 differential equations of rocket movement /Subsystem7 ==
  f/A : Inport
  Bus Selector : BusSelector  OutputSignals=signal1.signal5.signal1.Q,signal1.signal5.signal1.R,signal1.signal5.signal1.phi
  MATLAB Function : MATLAB Function  TreatAsAtomicUnit=on
  theta_dot : Outport
  wires:
  MATLAB Function/1(theta_dot) -> theta_dot/1
  f/A/1 -> Bus Selector/1
  Bus Selector/1 -> MATLAB Function/1(Q)  "<Q>"
  Bus Selector/2 -> MATLAB Function/2(R)  "<R>"
  Bus Selector/3 -> MATLAB Function/3(phi)  "<phi>"

== system simulation_model/Missile dynamics model/12 differential equations of rocket movement /Subsystem8 ==
  f/A : Inport
  Bus Selector : BusSelector  OutputSignals=signal1.signal5.signal1.Q,signal1.signal5.signal1.R,signal1.signal5.signal1.phi,signal1.signal5.signal1.theta
  MATLAB Function : MATLAB Function  TreatAsAtomicUnit=on
  psi_dot : Outport
  wires:
  Bus Selector/3 -> MATLAB Function/3(phi)  "<phi>"
  Bus Selector/2 -> MATLAB Function/2(R)  "<R>"
  Bus Selector/1 -> MATLAB Function/1(Q)  "<Q>"
  f/A/1 -> Bus Selector/1
  MATLAB Function/1(psi_dot) -> psi_dot/1
  Bus Selector/4 -> MATLAB Function/4(theta)  "<theta>"
  ? -> ?

== system simulation_model/Missile dynamics model/12 differential equations of rocket movement /Subsystem9 ==
  f/A : Inport
  Bus Selector : BusSelector  OutputSignals=signal1.signal5.signal1.U,signal1.signal5.signal1.V,signal1.signal5.signal1.W,signal1.signal5.signal1.theta,signal1.signal5.signal1.phi,signal1.signal5.signal1.psi
  MATLAB Function : MATLAB Function  TreatAsAtomicUnit=on
  x_dot : Outport
  wires:
  f/A/1 -> Bus Selector/1
  Bus Selector/1 -> MATLAB Function/1(U)  "<U>"
  Bus Selector/2 -> MATLAB Function/2(V)  "<V>"
  Bus Selector/3 -> MATLAB Function/3(W)  "<W>"
  Bus Selector/4 -> MATLAB Function/4(theta)  "<theta>"
  Bus Selector/5 -> MATLAB Function/5(phi)  "<phi>"
  Bus Selector/6 -> MATLAB Function/6(psi)  "<psi>"
  MATLAB Function/1(x_dot) -> x_dot/1

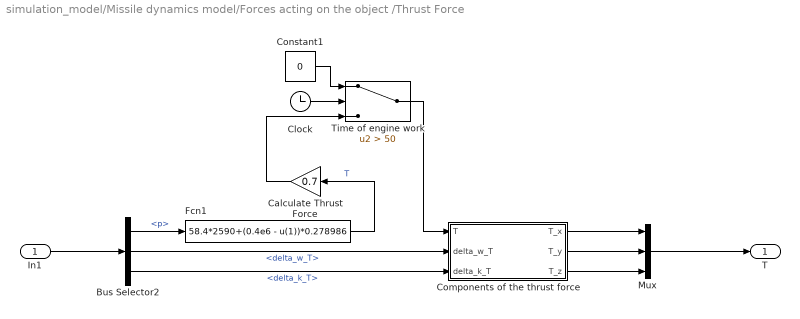
== system simulation_model/Missile dynamics model/Forces acting on the object /Thrust Force ==
  In1 : Inport
  Bus Selector2 : BusSelector  OutputSignals=signal5.signal2.signal2.p,delta_w_T,delta_k_T
  Calculate Thrust Force : Gain  Gain=0.7
  Clock : Clock
  Components of the thrust force : MATLAB Function  TreatAsAtomicUnit=on
  Constant1 : Constant  Value=0
  Fcn1 : Fcn  Expr=58.4*2590+(0.4e6 - u(1))*0.278986
  Mux : Mux  Inputs=3
  "Time of engine work " : Switch  Criteria=u2 > Threshold  Threshold=50  SaturateOnIntegerOverflow=off  InputSameDT=off
  T : Outport
  wires:
  Clock/1 -> "Time of engine work "/2
  Fcn1/1 -> Calculate Thrust Force/1  "T"
  "Time of engine work "/1 -> Components of the thrust force/1(T)
  Constant1/1 -> "Time of engine work "/1
  Bus Selector2/1 -> Fcn1/1  "<p>"
  Calculate Thrust Force/1 -> "Time of engine work "/3
  In1/1 -> Bus Selector2/1
  Mux/1 -> T/1
  Bus Selector2/2 -> Components of the thrust force/2(delta_w_T)  "<delta_w_T>"
  Bus Selector2/3 -> Components of the thrust force/3(delta_k_T)  "<delta_k_T>"
  Components of the thrust force/2(T_y) -> Mux/2
  Components of the thrust force/1(T_x) -> Mux/1
  Components of the thrust force/3(T_z) -> Mux/3

== matlab function simulation_model/Missile dynamics model/Forces acting on the object /Thrust Force/Components of the thrust force ==
  data: T input; T_x output; delta_w_T input; delta_k_T input; T_y output; T_z output
%% function which calculates Components of the thrust force
% 
% Inputs:
% T - Thrust force [N]
% delta_w_T - deflection of thrust force in axis Z [rad]
% delta_k_T - deflection of thrust force in axis Y [rad]
%
% Outputs:
% T_x - Thrust force in axis X [N]
% T_y - Thrust force in axis Y [N]
% T_z - Thrust force in axis Z [N]


function [T_x, T_y, T_z] = fcn(T, delta_w_T, delta_k_T)

T_y = T*sin(delta_k_T);
T_z = T*sin(delta_w_T);
T_x = sqrt(T^2 - T_y^2 - T_z^2);

== matlab function simulation_model/Missile dynamics model/Moments acting on the object/dynamic moment of force ==
  data: M_dm output; U input; W input; V input; Q input; R input; rho input; C_mq input
%% function which calculates Components of the aerodynamic dynamic moment
% 
% Inputs:
% U - velocity about x body axis [m/s]
% V - velocity about y body axis [m/s]
% W - velocity about z body axis [m/s]
% Q - pitch rate [ras/s]
% R - yaw rate [rad/s]
% rho - air density [kg/m^3]
% C_mq - Pitch damping coefficient
%
% Outputs:
% M_dm - Dynamic erodynamic moment [N*m]

function M_dm = fcn(U, W, V, Q, R, rho, C_mq)

% calculate cross-sectional area
S = pi*(0.92/2)^2;

% diameter of rocket
d = 0.92;

% calculate the absolute value of velocity
Vaer_bezwzgl = sqrt(U^2 + V^2 + W^2);

% calculate aerodynamic dynamic moment
M_dm_y = C_mq*(Q*d/Vaer_bezwzgl)*0.5*rho*Vaer_bezwzgl^2*S*d;
M_dm_z = C_mq*(R*d/Vaer_bezwzgl)*0.5*rho*Vaer_bezwzgl^2*S*d;

% vector aerodynamic dynamic moment
M_dm = [0; M_dm_y; M_dm_z];

% multiply aerodynamic dynamic moment by constans
M_dm = 4.*M_dm;

== matlab function simulation_model/Missile dynamics model/12 differential equations of rocket movement /Subsystem/MATLAB Function ==
  data: F input; U_dot output; m input; W input; Q input; V input; R input
%% function which calculates derivative of velocity about x body axis
% 
% Inputs:
% F - applied forces vector [N]
% m - mass of rocket [kg]
% W - velocity about z body axis [m/s]
% Q - pitch rate [ras/s] 
% V - velocity about y body axis [m/s]
% R - yaw rate [rad/s]
% Outputs:
% U_dot - derivative of velocity about x body axis [m/s^2]


function U_dot = fcn(F, m, W, Q, V, R)

U_dot = (F(1)+m*(R*V-Q*W))/m;

== matlab function simulation_model/Missile dynamics model/12 differential equations of rocket movement /Subsystem1/MATLAB Function ==
  data: F input; V_dot output; U input; R input; W input; P input; m input
%% function which calculates derivative of velocity about y body axis
% 
% Inputs:
% F - applied forces vector [N]
% U - velocity about x body axis [m/s] 
% R - yaw rate [rad/s]
% W - velocity about z body axis [m/s]
% P - roll rate [rad/s]
% m - mass of rocket [kg]
%
% Outputs:
% V_dot - derivative of velocity about y body axis [m/s^2]


function V_dot = fcn(F, U, R, W, P, m)
V_dot = zeros(1,1);

V_dot = (F(2)+m.*(P.*W-R.*U))./m;

== matlab function simulation_model/Missile dynamics model/12 differential equations of rocket movement /Subsystem2/MATLAB Function ==
  data: F input; W_dot output; m input; U input; Q input; V input; P input
%% function which calculates derivative of velocity about z body axis
% 
% Inputs:
% F - applied forces vector [N]
% m - mass of rocket [kg]
% U - velocity about x body axis [m/s^2] 
% Q - pitch rate [rad/s]
% V - velocity about y body axis [m/s]
% P - roll rate [rad/s]
%
% Outputs:
% W_dot - derivative of velocity about z body axis [m/s^2]

function W_dot = fcn(F, m, U, Q, V, P)
W_dot = zeros(1,1);

W_dot = (F(3)+m.*(Q.*U-P.*V))./m;

== matlab function simulation_model/Missile dynamics model/12 differential equations of rocket movement /Subsystem3/MATLAB Function ==
  data: M input; P_dot output; I_x input
%% function which calculates derivative of roll rate
% 
% Inputs:
% M - Aerodynamic moment [N*m] 
% I_x - moment of inertia Ix [kg*m^2]
%
% Outputs:
% P_dot - derivative of roll rate [rad/s^2]


function P_dot = fcn(M, I_x)

P_dot = M(1)/I_x;

== matlab function simulation_model/Missile dynamics model/12 differential equations of rocket movement /Subsystem4/MATLAB Function ==
  data: M input; Q_dot output; P input; R input; I input; I_x input
%% function which calculates derivative of pitch rate 
% 
% Inputs:
% M - Aerodynamic moment [N*m] 
% P - roll rate [rad/s]
% R - yaw rate [rad/s]
% I - moments of inertia Iy and Iz [kg*m^2]
% I_x - moment of inertia Ix [kg*m^2]
%
% Outputs:
% Q_dot - derivative of pitch rate [rad/s^2]


function Q_dot = fcn(M, P, R, I, I_x)
Q_dot = zeros(1,1);

Q_dot = (M(2)+P*R*(I-I_x))/I;

== matlab function simulation_model/Missile dynamics model/12 differential equations of rocket movement /Subsystem5/MATLAB Function ==
  data: M input; R_dot output; P input; Q input; I input; I_x input
%% function which calculates derivative of yaw rate
% 
% Inputs:
% M - Aerodynamic moment [N*m] 
% P - roll rate [rad/s]
% Q - pitch rate [rad/s]
% I - moments of inertia Iy and Iz [kg*m^2]
% I_x - moment of inertia Ix [kg*m^2]
%
% Outputs:
% R_dot - derivative of yaw rate [rad/s^2]

function R_dot = fcn(M, P, Q, I, I_x)
R_dot = zeros(1,1);

R_dot = (M(3)+P*Q*(I_x-I))/I;

== matlab function simulation_model/Missile dynamics model/12 differential equations of rocket movement /Subsystem6/MATLAB Function ==
  data: P input; Q input; phi_dot output; phi input; R input; theta input
%% function which calculates derivative of roll angle [rad]
% 
% Inputs:
% P - roll rate [rad/s] 
% Q - pitch rate [rad/s]
% phi - roll angle [rad]
% R - yaw rate [rad/s]
% theta - pitch angle [rad]
%
% Outputs:
% phi_dot - derivative of yaw rate [rad/s]

function phi_dot = fcn(P, Q, phi, R, theta)

phi_dot = P + (Q*sin(phi)+R*cos(phi))*tan(theta);
phi_dot = 0; % physical assumption

== matlab function simulation_model/Missile dynamics model/12 differential equations of rocket movement /Subsystem7/MATLAB Function ==
  data: Q input; R input; theta_dot output; phi input
%% function which calculates derivative of pitch  angle [rad]
% 
% Inputs:
% Q - pitch rate [rad/s]
% R - yaw rate [rad/s]
% phi - roll angle [rad]
%
% Outputs:
% theta_dot - derivative of pitch  rate [rad/s]


function theta_dot = fcn(Q, R, phi)

theta_dot = Q*cos(phi) - R*sin(phi);

== matlab function simulation_model/Missile dynamics model/12 differential equations of rocket movement /Subsystem8/MATLAB Function ==
  data: Q input; R input; psi_dot output; phi input; theta input
%% function which calculates derivative of yaw angle [rad]
% 
% Inputs:
% Q - pitch rate [rad/s]
% R - yaw rate [rad/s]
% phi - roll angle [rad]
% theta - pitch angle [rad]
%
% Outputs:
% psi_dot - derivative of yaw rate [rad/s]


function psi_dot = fcn(Q, R, phi, theta)

psi_dot = (Q*sin(phi) + R*cos(phi))/cos(theta);

== matlab function simulation_model/Missile dynamics model/12 differential equations of rocket movement /Subsystem9/MATLAB Function ==
  data: U input; V input; W input; x_dot output; theta input; phi input; psi input
%% function which calculates derivative of x object coordinates [m]
% 
% Inputs:
% U - velocity about x body axis [m/s] 
% V - velocity about y body axis [m/s]
% W - velocity about z body axis [m/s]
% theta - pitch angle [rad]
% phi - roll angle [rad]
% psi - yaw angle [rad]
%
% Outputs:
% x_dot - derivative of x object coordinates [m]


function x_dot = fcn(U, V, W, theta, phi, psi)

x_dot = U*cos(psi)*cos(theta) + V*(cos(psi)*sin(theta)*sin(phi)-sin(psi)*cos(phi)) + W*(cos(psi)*sin(theta)*cos(phi)+sin(psi)*sin(phi));

== matlab function simulation_model/Missile dynamics model/12 differential equations of rocket movement /Subsystem10/MATLAB Function ==
  data: U input; V input; W input; y_dot output; theta input; phi input; psi input
%% function which calculates derivative of y object coordinates [m]
% 
% Inputs:
% U - velocity about x body axis [m/s] 
% V - velocity about y body axis [m/s]
% W - velocity about z body axis [m/s]
% theta - pitch angle [rad]
% phi - roll angle [rad]
% psi - yaw angle [rad]
%
% Outputs:
% y_dot - derivative of y object coordinates [m]

function y_dot = fcn(U, V, W, theta, phi, psi)

y_dot = U*sin(psi)*cos(theta) + V*(sin(psi)*sin(theta)*sin(phi)+cos(psi)*cos(phi)) + W*(sin(psi)*sin(theta)*cos(phi)-cos(psi)*sin(phi));

== matlab function simulation_model/Missile dynamics model/12 differential equations of rocket movement /Subsystem11/MATLAB Function ==
  data: U input; V input; W input; z_dot output; theta input; phi input
%% function which calculates derivative of z object coordinates [m]
% 
% Inputs:
% U - velocity about x body axis [m/s] 
% V - velocity about y body axis [m/s]
% W - velocity about z body axis [m/s]
% theta - pitch angle [rad]
% phi - roll angle [rad]
%
% Outputs:
% z_dot - derivative of z object coordinates [m]

function z_dot = fcn(U, V, W, theta, phi)

z_dot = -U*sin(theta) + V*cos(theta)*sin(phi) + W*cos(theta)*cos(phi);

== matlab function simulation_model/Missile dynamics model/Moments acting on the object/static moment of force ==
  data: M_st2 output; T input; C_Na_kadl input; M_st output; rho input; W input; V input; U input; n_p input; C_Na_ster input; x_sm input; alfa input; beta input; C_ma input; alfa_t input; x_sp_kadl input; x_sp_ster input; delta_w input; delta_k input
%% function which calculates Components of the aerodynamic static moment
% 
% Inputs:
% T - thrust force [N]
% C_Na_kadl - Derivative of normal force coefficient after sin\alpha for monocoque
% rho - air density [kg/m^3]
% U - velocity about x body axis [m/s]
% V - velocity about y body axis [m/s]
% W - velocity about z body axis [m/s]
% n_p - unit vector
% C_Na_ster - Derivative of normal force coefficient after sin\alpha for fins
% x_sm - coordinate of the center of gravity [m]
% alfa - angle of attack [rad]
% beta - angle of sideslip [rad] 
% C_ma - Derivative after pitch moment coefficient slope after sin\alpha
% alfa_t - total angle of attack [rad]
% x_sp_kadl - coordinate center of pressure for monocoque [m]
% x_sp_ster - coordinate center of pressure for fins [m]
% delta_w - deflection of fins in axis Z [rad]
% delta_k - deflection of fins in axis Y [rad]
% 
% Outputs:
% [M_st, M_st2] - Static aerodynamic moments [N*m]


function [M_st2, M_st] = fcn(T, C_Na_kadl, rho, W, V, U, n_p, C_Na_ster, x_sm, alfa, beta, C_ma, alfa_t, x_sp_kadl, x_sp_ster, delta_w, delta_k)
M_st = zeros(3,1);
M_st2 = zeros(3,1);

% calculate cross-sectional area
S = pi*(0.92/2)^2;

% diameter of rocket
d = 0.92;

% length of rocket
L = 7.28;

% calculate the absolute value of velocity
Vaer_bezwzgl = sqrt(U^2 + V^2 + W^2);

% calculate aerodynamic coefficients of izolated elements
C_N_y_kadl = C_Na_kadl*sin(beta);
C_N_y_ster = C_Na_ster*sin(beta+delta_k); 
C_N_z_kadl = C_Na_kadl*cos(beta)*sin(alfa);
C_N_z_ster = C_Na_ster*cos(beta)*sin(alfa+delta_w);

% calculate aerodynamic coefficients
C_m_p_y = C_N_z_kadl*(x_sm-x_sp_kadl) + C_N_z_ster*(x_sm-x_sp_ster);
C_m_p_z = C_N_y_kadl*(x_sm-x_sp_kadl) + C_N_y_ster*(x_sm-x_sp_ster);

% calculate aerodynamic moments
M_p_y = C_m_p_y*0.5*rho*Vaer_bezwzgl^2*S*d;
M_p_z = C_m_p_z*0.5*rho*Vaer_bezwzgl^2*S*d;

% components of the thrust vector
T_y = T(2);
T_z = T(3);

% torque from the thrust force
M_T = [0; T_z*(x_sm-L); T_y*(x_sm-L)];

% vector of aerodynamic moments
M_p = [0; M_p_y; -M_p_z];

% calculate aerodynamic moments by unit vector
M_p2 = C_ma*sin(alfa_t)*0.5*rho*Vaer_bezwzgl^2*S*d*n_p;

% calculate aerodynamic static moment
M_st = M_p + M_T;
M_st2 = M_p2 + M_T;

== matlab function simulation_model/Rocket control model/thrust vector cotrol ==
  data: theta input; psi input; alfa input; beta input; gamma_p input; gamma2_p input; t input; K_w_T output; K_k_T output
%% function which calculates thrust vectoring control commands
% 
% Inputs:
% theta - pitch angle [rad]
% psi - yaw angle [rad]
% alfa - angle of attack [rad]
% beta -  angle of sideslip [rad]
% gamma_p - programmable pith angle [rad]
% gamma2_p - programmable yaw angle [rad]
% t - time of flight [s]
%
% Outputs:
% K_w_T - command control of thrust vectoring in axis Z
% K_k_T - command control of thrust vectoring in axis Y


function [K_w_T, K_k_T] = fcn(theta, psi, alfa, beta, gamma_p, gamma2_p, t)
k = -1.3;
kat = 0.3;
gamma = theta - alfa;
gamma2 = psi - beta;

if t < 9
    gamma_p = deg2rad(90);
end

if t < 50
    u1 = gamma_p - (gamma);
    u2 = gamma2_p - (gamma2);

    

    if u1 < 0 
        K_w_T = k*u1;
        if K_w_T > kat
            K_w_T = deg2rad(kat);
        else
            K_w_T = deg2rad(K_w_T);
        end
         
    elseif u1 > 0 
        K_w_T = k*u1;
        if K_w_T < kat
            K_w_T = deg2rad(-kat);
        else
            K_w_T = deg2rad(K_w_T);
        end
    else
        K_w_T = 0;
    end

    if u2 < 0 && t > 10
        K_k_T = k*u2;
        if K_k_T > kat
            K_k_T = deg2rad(kat);
        else
            K_k_T = deg2rad(K_k_T);
        end
    elseif u2 > 0 && t > 10
        K_k_T = k*u2;
        if K_k_T < kat
            K_k_T = deg2rad(-kat);
        else
            K_k_T = deg2rad(K_k_T);
        end
    else
        K_k_T = 0;
    end
else
    K_w_T = 0;
    K_k_T = 0;
end
% K_k_T = 0;

== matlab function simulation_model/Parameters of rocket 9M723 and atmosphere model/Unit vectors and movement angles ==
  data: U input; n_x output; n_V output; n_p output; n_N output; alfa_t output; alfa output; beta output; V input; W input
%% function which calculates Unit vectors and movement angles
% 
% Inputs:
% U - velocity about x body axis [m/s]
% V - velocity about y body axis [m/s]
% W - velocity about z body axis [m/s]
%
% Outputs:
% n_x, n_V, n_p, n_N - unit vectors used to calculate forces and moments
% alfa_t - total angle of attack [rad]
% alfa - angle of attack [rad]
% beta - angle of sideslip [rad]

function [n_x, n_V, n_p, n_N, alfa_t, alfa, beta] = fcn(U, V, W)

% calculate velocity
Vaer = [U, V, W];
Vaer_bezwzgl = sqrt(Vaer(1)^2 + Vaer(2)^2 + Vaer(3)^2);

% define unit vector
n_x = [1 0 0]';

% calculate unit vectors
n_V = [Vaer(1)/Vaer_bezwzgl Vaer(2)/Vaer_bezwzgl Vaer(3)/Vaer_bezwzgl]';
% preventing division by zero
if n_V(3) == 0
    n_V(3) = 0.0000000000001;
end

n_p = 1/(sqrt(n_V(3)^2+n_V(2)^2))*[0; n_V(3); -n_V(2)];

n_N = [n_x(2)*n_p(3)-n_x(3)*n_p(2)
      n_x(3)*n_p(1)-n_x(1)*n_p(3)
      n_x(1)*n_p(2)-n_x(2)*n_p(1)] ...
      /sqrt((n_x(2)*n_p(3)-n_x(3)*n_p(2))^2 ...
      + (n_x(3)*n_p(1)-n_x(1)*n_p(3))^2 ... 
      + (n_x(1)*n_p(2)-n_x(2)*n_p(1))^2);

% calculate  movement angles
alfa_t = acos(n_V(1));
alfa = atan(Vaer(3)/Vaer(1));
beta = asin(Vaer(2)/Vaer_bezwzgl);
